simulink model "distff"  (Simulink 3.00)
settings: Solver=ode45  SolverMode=SingleTasking  StartTime=0.0  StopTime=15  MaxStep=0.01  RelTol=1e-3  AbsTol=1e-3
settings Model: TimeSaveName=t  SaveOutput=off

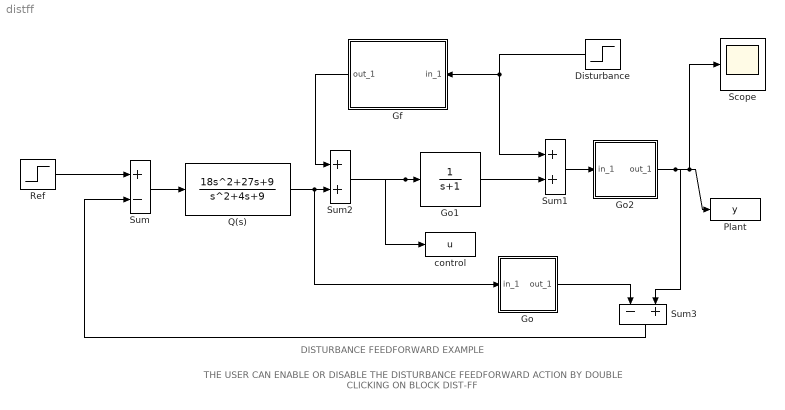
== system distff ==
  note: THE USER CAN ENABLE OR DISABLE THE DISTURBANCE FEEDFORWARD ACTION
      |  BY DOUBLE CLICKING ON BLOCK DIST-FF
  note: DISTURBANCE FEEDFORWARD EXAMPLE
  Disturbance : Step  Orientation=left  Time=5  Before=0  After=1  SampleTime=0
  Gf : Subsystem  Orientation=left  mask(Disturbance feedforward){@1=0, @2=[-1 -1], @3=[0.2 1]}
      mask prompts: @1 "ON (1) or OFF (0):"; @2 "numerator of Gf:"; @3 "denominator of Gf"
      mask help: Disturbance feedforward
      mask init:
      | K=@1;ngf=@2;dgf=@3;
      mask Display: disp('DIST-FF')
  Go : Subsystem
      mask Type: Go
      mask Display: disp('Go(s)')
  Go1 : TransferFcn  Numerator=[1]  Denominator=[1 1]
      mask Type: Go1
      mask Display: disp('Go1(s)')
  Go2 : Subsystem
      mask Type: Go2
      mask Display: disp('Go2(s)')
  Plant : ToWorkspace  VariableName=y  SampleTime=0  SaveFormat=Matrix
      settings: Buffer=6000
  Q(s) : TransferFcn  Numerator=[18 27 9]  Denominator=[1 4 9]
  Ref : Step  Time=1  Before=0  After=1  SampleTime=0
  Scope : Scope
      settings: TickLabels=on  TimeRange=15.000000  YMin=-1.500000  YMax=1.500000  SaveToWorkspace=off  SaveName=ScopeData  DataFormat=Matrix
  Sum : Sum  Inputs=+-  SaturateOnIntegerOverflow=on
  Sum1 : Sum  Inputs=++  SaturateOnIntegerOverflow=on
  Sum2 : Sum  Inputs=++  SaturateOnIntegerOverflow=on
  Sum3 : Sum  Orientation=down  Inputs=-+  SaturateOnIntegerOverflow=on
  control : ToWorkspace  VariableName=u  SampleTime=0  SaveFormat=Matrix
      settings: Buffer=6000
  wires:
  Sum/1 -> Q(s)/1
  Go1/1 -> Sum1/2
  Sum1/1 -> Go2/1(in_1)
  Go/1(out_1) -> Sum3/1
  Sum3/1 -> Sum/2
  Ref/1 -> Sum/1
  Q(s)/1 -> Sum2/2, Go/1(in_1)
  Go2/1(out_1) -> Plant/1, Sum3/2, Scope/1
  Sum2/1 -> Go1/1, control/1
  Gf/1(out_1) -> Sum2/1
  Disturbance/1 -> Sum1/1, Gf/1(in_1)

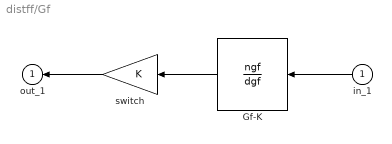
== system distff/Gf ==
  in_1 : Inport  Orientation=left  Port=1  PortWidth=-1  SampleTime=-1  DataType=auto
      settings: SignalType=auto
  Gf-K : TransferFcn  Orientation=left  Numerator=ngf  Denominator=dgf
  switch : Gain  Orientation=left  Gain=K  SaturateOnIntegerOverflow=on
  out_1 : Outport  Orientation=left  Port=1  InitialOutput=0
  wires:
  Gf-K/1 -> switch/1
  switch/1 -> out_1/1
  in_1/1 -> Gf-K/1

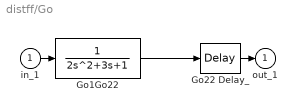
== system distff/Go ==
  in_1 : Inport  Port=1  PortWidth=-1  SampleTime=-1  DataType=auto
      settings: SignalType=auto
  Go1Go22 : TransferFcn  Numerator=[1]  Denominator="[2 3  1]"
  Go22 Delay_ : TransportDelay  DelayTime=1  InitialInput=0  BufferSize=1024
  out_1 : Outport  Port=1  InitialOutput=0
  wires:
  Go1Go22/1 -> Go22 Delay_/1
  in_1/1 -> Go1Go22/1
  Go22 Delay_/1 -> out_1/1

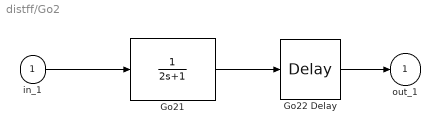
== system distff/Go2 ==
  in_1 : Inport  Port=1  PortWidth=-1  SampleTime=-1  DataType=auto
      settings: SignalType=auto
  Go21 : TransferFcn  Numerator=[1]  Denominator=[2 1]
  Go22 Delay : TransportDelay  DelayTime=1  InitialInput=0  BufferSize=1024
  out_1 : Outport  Port=1  InitialOutput=0
  wires:
  Go21/1 -> Go22 Delay/1
  Go22 Delay/1 -> out_1/1
  in_1/1 -> Go21/1
